simulink model "inverse_model"  (R2019b)
settings: Solver=VariableStepAuto  StartTime=0.0  StopTime=10.0  RelTol=1e-4
values from neighbouring files (symbols this model uses):
  f = 2.0    (= 2)    [parameters.m]
  F = [0.1, 0 ... (first row only)    [parameters.m]
  K_d = [10 0; 0 10]    [parameters.m]
  K_p = [25 0; 0 25]    [parameters.m]
settings Model: Creator=stephhan  LastModifiedBy=stephhan

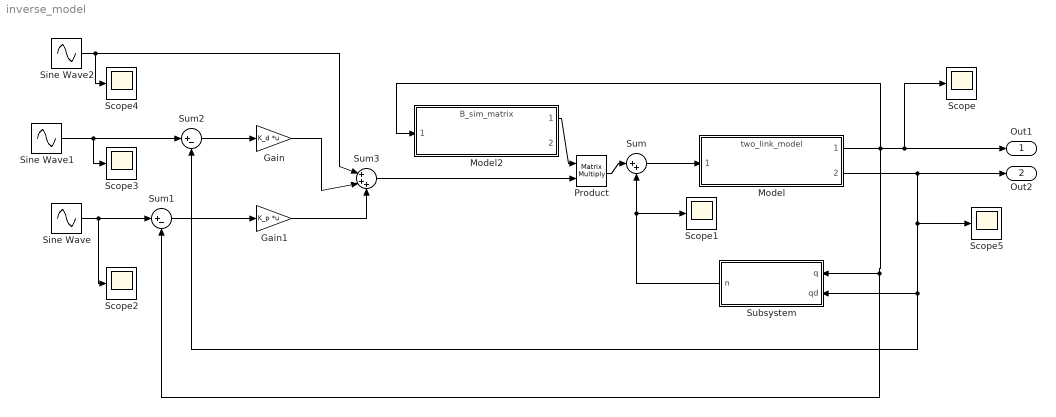
== system inverse_model ==
  Gain : Gain  Gain=K_d  Multiplication=Matrix(K*u)
  Gain1 : Gain  Gain=K_p  Multiplication=Matrix(K*u)
  Model : ModelReference  ModelNameDialog=two_link_model  SimulationMode=Normal  ModelReferenceVersion=1.3
  Model2 : ModelReference  ModelNameDialog=B_sim_matrix  SimulationMode=Normal  ModelReferenceVersion=1.6
  Product : Product  Multiplication=Matrix(*)
  Scope{,1..5} (6 alike) : Scope
  Sine Wave : Sin  Frequency=[2*pi*f;2*pi*f]  SampleTime=0
  Sine Wave1 : Sin  Amplitude=2*pi*f  Frequency=[2*pi*f;2*pi*f]  Phase=pi/2  SampleTime=0
  Sine Wave2 : Sin  Amplitude=-4*pi*pi*f*f  Frequency=[2*pi*f;2*pi*f]  SampleTime=0
  Subsystem : Subsystem
  Sum : Sum  Inputs=|++
  Sum1 : Sum  Inputs=|+-
  Sum2 : Sum  Inputs=|+-
  Sum3 : Sum  Inputs=|+++
  Out1 : Outport
  Out2 : Outport  Port=2
  wires:
  Model/1 -> Model2/1, Subsystem/1(q), Sum1/2, Scope/1, Out1/1
  Model/2 -> Scope5/1, Subsystem/2(qd), Sum2/2, Out2/1
  Sum/1 -> Model/1
  Subsystem/1(n) -> Scope1/1, Sum/2
  Sum3/1 -> Product/2
  Sum2/1 -> Gain/1
  Sum1/1 -> Gain1/1
  Gain1/1 -> Sum3/3
  Gain/1 -> Sum3/2
  Sine Wave/1 -> Scope2/1, Sum1/1
  Sine Wave1/1 -> Scope3/1, Sum2/1
  Sine Wave2/1 -> Scope4/1, Sum3/1
  Product/1 -> Sum/1
  Model2/1 -> Product/1

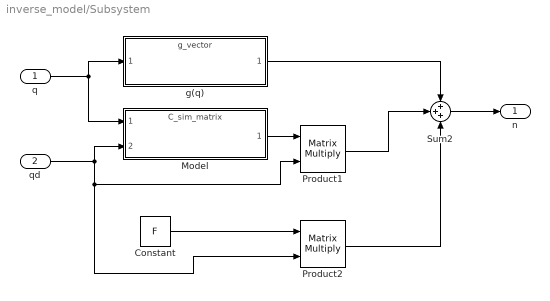
== system inverse_model/Subsystem ==
  q : Inport  PortDimensions=2
  qd : Inport  Port=2  PortDimensions=2
  Constant : Constant  Value=F
  Model : ModelReference  ModelNameDialog=C_sim_matrix.slx  SimulationMode=Normal  ModelReferenceVersion=1.2
  Product1 : Product  Multiplication=Matrix(*)
  Product2 : Product  Multiplication=Matrix(*)
  Sum2 : Sum  Inputs=+++
  g(q) : ModelReference  ModelNameDialog=g_vector.slx  SimulationMode=Normal  ModelReferenceVersion=1.8
  n : Outport
  wires:
  Sum2/1 -> n/1
  Product2/1 -> Sum2/3
  g(q)/1 -> Sum2/1
  Model/1 -> Product1/1
  qd/1 -> Model/2, Product1/2, Product2/2
  q/1 -> Model/1, g(q)/1
  Constant/1 -> Product2/1
  Product1/1 -> Sum2/2
